simulink model "model_nielin"  (R2017a)
settings: Solver=ode15s  StartTime=0.0  StopTime=10  FixedStep=1e-3  MaxStep=1e-3  RelTol=1e-3
values from neighbouring files (symbols this model uses):
  a0 = m*v*T0/M    (= 6)    [model.m]
  a1 = m*v/M    (= 0.3)    [model.m]
  a2 = ((n+1)*gs*cs*Tp)/(M*c)    (= 15)    [model.m]
  a3 = ((n+1)*gs*cs)/(M*c)    (= 0.01)    [model.m]
  dq = 1    [model.m]
  qpracy = (B*(Tpracy-T0))/(A*(Tp-Tpracy))    (= 33.4285714286)    [model.m]    (also in stat.m = 0:0.01:150)
  Tpracy = 800    [model.m]    (also in stat.m = (A*Tp*qpracy+B*T0)./(A*qpracy+B))
settings Model: Creator=Piotr  LastModifiedBy=Piotr

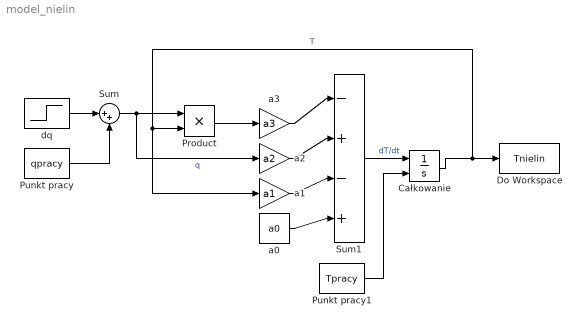
== system model_nielin ==
  " dq" : Step  Time=0  After=dq  SampleTime=0
  Całkowanie : Integrator  InitialConditionSource=external  InitialCondition=Tpracy
  Do Workspace : ToWorkspace  VariableName=Tnielin  SaveFormat=Timeseries  SampleTime=1e-3
  Product : Product
  Punkt pracy : Constant  Value=qpracy
  Punkt pracy1 : Constant  Value=Tpracy
  Sum : Sum  Inputs=|++
  Sum1 : Sum  Inputs=|-+-+
  a0 : Constant  Value=a0
  a1 : Gain  Gain=a1
  a2 : Gain  Gain=a2
  a3 : Gain  Gain=a3
  wires:
  " dq"/1 -> Sum/1
  Punkt pracy/1 -> Sum/2
  Sum/1 -> a2/1, Product/1  "q"
  Product/1 -> a3/1
  a3/1 -> Sum1/1
  Sum1/1 -> Całkowanie/1  "dT/dt"
  Całkowanie/1 -> Do Workspace/1, a1/1, Product/2  "T"
  a2/1 -> Sum1/2
  a1/1 -> Sum1/3
  a0/1 -> Sum1/4
  Punkt pracy1/1 -> Całkowanie/2
